simulink model "gm_sampleModel1438_4_sub"  (R2023a)
settings: Solver=VariableStepAuto  StartTime=0.0  StopTime=10.0  RelTol=1e-3
libraries: simulink x1, hdlsllib x1
settings Model: Creator=user1  LastModifiedBy=user1
settings OptimizationCC: BlockReduction=off  ConditionallyExecuteInputs=off
settings DebuggingCC: InheritedTsInSrcMsg=none

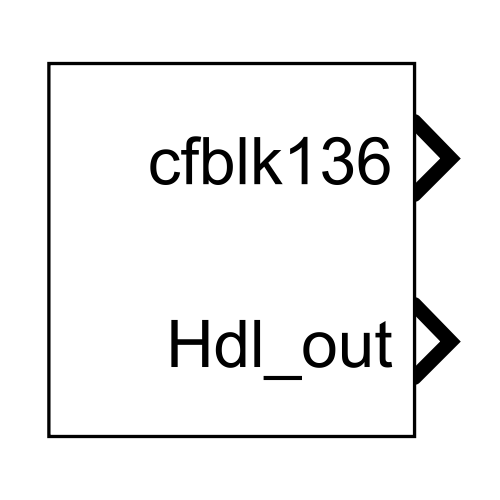
[thumbnail: Simulink's stored preview of the top-level diagram]
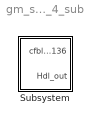
== system gm_sampleModel1438_4_sub ==
  Subsystem : Subsystem

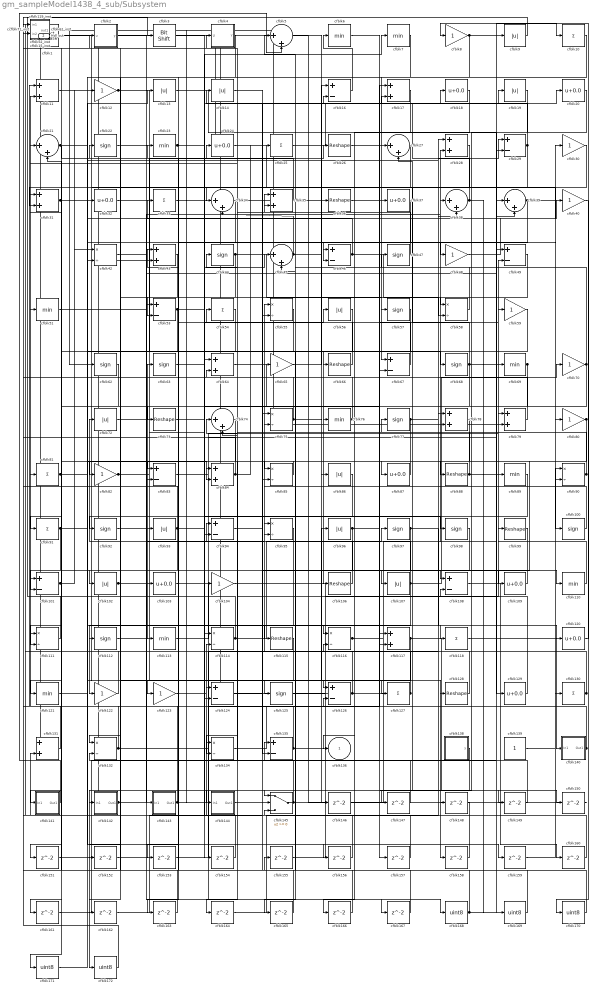
== system gm_sampleModel1438_4_sub/Subsystem ==
  cfblk1 : simulink/Logic and Bit Operations/Detect Decrease  vinit=0.0  OutDataTypeStr=uint8
      settings: LibrarySourceBlock=|
      | hdlsllib/Logic and Bit
      | Operations/Detect
      | Decrease
  cfblk{10,25,33,54,81,91,118,127,130} (9 alike) : Sum  Inputs=+  OutDataTypeStr=uint8
  cfblk{22,44,47,57,62..63,68,77,92,97..98,100,112,125} (14 alike) : Signum
  cfblk{16,29,46,49,53,67,83,94,101,108,124,126,135} (13 alike) : Sum  Inputs=+-  OutDataTypeStr=uint8
  cfblk{9,13..14,19,56,72,86,93,96,102,107} (11 alike) : Abs  OutDataTypeStr=uint8  SaturateOnIntegerOverflow=off
  cfblk{18,20,24,32,37,87,103,109,120,129} (10 alike) : Bias  Bias=0.0  SaturateOnIntegerOverflow=off
  cfblk{8,12,30,40,48,59,65,70,80,82,104,122..123} (13 alike) : Gain  OutDataTypeStr=uint8
  cfblk105_inst : Subsystem
  cfblk{26,36,66,73,88,99,106,115,128} (9 alike) : Reshape
  cfblk{11,17,28,31,35,43,64,78..79,84,117,131} (12 alike) : Sum  OutDataTypeStr=uint8
  cfblk{6..7,23,51,69,76,89,110,113,121} (10 alike) : MinMax  OutDataTypeStr=uint8
  cfblk{42,55,58,75,85,90,95,111,114,116,132,134} (12 alike) : Product  Inputs=*/  OutDataTypeStr=uint8  RndMeth=Zero  SaturateOnIntegerOverflow=on
  cfblk119_inst : Subsystem
  cfblk138 : Subsystem  mask(Counter Free-Running){NumBits=double(16), tsamp=double(-1)}
      mask prompts: NumBits "Simulink:masks:NumberOfBits_MP"; tsamp "Simulink:masks:SampleTime_MP"
      mask help: Simulink:masks:CounterFreeRunning_MD
  cfblk139 : Constant  OutDataTypeStr=uint8  SampleTime=-1
  cfblk140 : Subsystem
  cfblk141 : Subsystem
  cfblk142 : Subsystem
  cfblk143 : Subsystem
  cfblk144 : Subsystem
  cfblk145 : Switch  OutDataTypeStr=uint8  SaturateOnIntegerOverflow=off  InputSameDT=off
  cfblk{146..167} (22 alike) : Delay  SampleTime=1
  cfblk15_inst : Subsystem
  cfblk{168..172} (5 alike) : DataTypeConversion  OutDataTypeStr=uint8  SaturateOnIntegerOverflow=off  RndMeth=Floor
  cfblk2 : Subsystem  mask(Compare To Zero){relop=<=, OutDataTypeStr=uint8, ZeroCross=on}
      mask prompts: relop "Simulink:masks:Operator_MP"; OutDataTypeStr "Simulink:masks:OutputDataType_MP"; ZeroCross "Simulink:masks:EnableZerocrossingDetection_MP"
      mask help: Simulink:masks:CompareToZero_MD
      mask init:
      | OutDataTypeStr = 'uint8';
      | ZeroCross = 'on';
      | blkName = 'sampleModel1438_4_sub/Subsystem/cfblk2';
      | relop = '<=';
      | setValue = 'fixdt(0, 8)';
      mask TypeOptions relop: == | ~= | < | <= | >= | >
      mask TypeOptions OutDataTypeStr: Simulink:masks:uint8 | Simulink:masks:boolean
      mask Callback ZeroCross: sl('zeroCrossEnable', gcbh);
      mask Display: disp([relop,' 0'])
  cfblk{5,21,27,34,38..39,45,74} (8 alike) : Sum  Inputs=|++  OutDataTypeStr=uint8
  cfblk3 : hdlsllib/Logic and Bit Operations/Bit Shift  mode=Shift Left Logical  N=0
  cfblk4 : Subsystem  mask(Detect Fall Nonpositive){vinit=double(0), InputProcessing=Elements as channels (sample based), OutDataTypeStr=uint8}
      mask prompts: vinit "Simulink:masks:InitialCondition_MP"; InputProcessing "Simulink:masks:InputProcessing_MP"; OutDataTypeStr "Simulink:masks:OutputDataType_MP"
      mask help: Simulink:masks:DetectFallNonpositive_MD
      mask init:
      | InputProcessing = 'Elements as channels (sample based)';
      | OutDataTypeStr = 'uint8';
      | vinit = double(0);
      mask TypeOptions InputProcessing: Simulink:masks:ColumnsAsChannelsFrameBased | Simulink:masks:ElementsAsChannelsSampleBased
      mask TypeOptions OutDataTypeStr: Simulink:masks:uint8 | Simulink:masks:boolean
      mask Display: fprintf('U <= 0\n&  NOT\nU/z <= 0')
  cfblk52_inst : Subsystem
  cfblk61_inst : Subsystem
  cfblk71_inst : Subsystem
  cfblk136 : Outport  OutDataTypeStr=uint8  SampleTime=1  VectorParamsAs1DForOutWhenUnconnected=off
  Hdl_out : Outport  Port=2  OutDataTypeStr=uint8  SampleTime=1
  wires:
  cfblk1/1 -> cfblk123/1
  cfblk10/1 -> cfblk67/1
  cfblk100/1 -> cfblk55/1
  cfblk101/1 -> cfblk32/1, cfblk42/1
  cfblk102/1 -> cfblk24/1, cfblk158/1
  cfblk103/1 -> cfblk167/1
  cfblk104/1 -> cfblk108/2
  cfblk105_inst/1(out1) -> cfblk143/1(In1)
  cfblk106/1 -> cfblk72/1
  cfblk107/1 -> cfblk75/2, cfblk70/1, cfblk122/1
  cfblk108/1 -> cfblk160/1
  cfblk109/1 -> cfblk108/1
  cfblk11/1 -> cfblk90/2
  cfblk110/1 -> cfblk49/2
  cfblk111/1 -> cfblk3/1
  cfblk112/1 -> cfblk63/1
  cfblk113/1 -> cfblk79/1
  cfblk114/1 -> cfblk97/1, cfblk11/2
  cfblk115/1 -> cfblk125/1
  cfblk116/1 -> cfblk39/1, cfblk28/2
  cfblk117/1 -> cfblk150/1, cfblk132/1
  cfblk118/1 -> cfblk140/1(In1)
  cfblk119_inst/1(out1) -> cfblk36/1
  cfblk12/1 -> cfblk93/1, cfblk106/1
  cfblk120/1 -> cfblk8/1
  cfblk121/1 -> cfblk28/1
  cfblk122/1 -> cfblk51/1
  cfblk123/1 -> cfblk114/2
  cfblk124/1 -> cfblk18/1
  cfblk125/1 -> cfblk99/1
  cfblk126/1 -> cfblk74/1, cfblk54/1
  cfblk127/1 -> cfblk95/1, Hdl_out/1
  cfblk128/1 -> cfblk61_inst/1(in1)
  cfblk129/1 -> cfblk64/2
  cfblk13/1 -> cfblk129/1
  cfblk130/1 -> cfblk74/2, cfblk45/2
  cfblk131/1 -> cfblk11/1
  cfblk132/1 -> cfblk78/1, cfblk119_inst/1(in1)
  cfblk134/1 -> cfblk37/1
  cfblk135/1 -> cfblk22/1, cfblk17/1
  cfblk138/1(y) -> cfblk172/1
  cfblk139/1 -> cfblk130/1
  cfblk14/1 -> cfblk75/1
  cfblk140/1(Out1) -> cfblk94/1, cfblk64/1
  cfblk141/1(Out1) -> cfblk5/2
  cfblk142/1(Out1) -> cfblk38/1, cfblk95/2
  cfblk143/1(Out1) -> cfblk126/2, cfblk81/1
  cfblk144/1(Out1) -> cfblk55/2
  cfblk145/1 -> cfblk96/1, cfblk14/1
  cfblk146/1 -> cfblk78/2
  cfblk147/1 -> cfblk132/2
  cfblk148/1 -> cfblk145/3
  cfblk149/1 -> cfblk35/1
  cfblk15_inst/1(out1) -> cfblk27/1
  cfblk150/1 -> cfblk1/1
  cfblk151/1 -> cfblk94/2
  cfblk152/1 -> cfblk85/2
  cfblk153/1 -> cfblk116/2
  cfblk154/1 -> cfblk131/2
  cfblk155/1 -> cfblk67/2
  cfblk156/1 -> cfblk105_inst/2(in2)
  cfblk157/1 -> cfblk124/1
  cfblk158/1 -> cfblk83/2
  cfblk159/1 -> cfblk90/1
  cfblk16/1 -> cfblk6/1
  cfblk160/1 -> cfblk52_inst/2(in2)
  cfblk161/1 -> cfblk39/2
  cfblk162/1 -> cfblk114/1
  cfblk163/1 -> cfblk31/1
  cfblk164/1 -> cfblk38/2
  cfblk165/1 -> cfblk43/1
  cfblk166/1 -> cfblk135/1
  cfblk167/1 -> cfblk145/2
  cfblk168/1 -> cfblk9/1, cfblk155/1
  cfblk169/1 -> cfblk2/1(u)
  cfblk17/1 -> cfblk166/1
  cfblk170/1 -> cfblk71_inst/1(in1)
  cfblk171/1 -> cfblk40/1
  cfblk172/1 -> cfblk71_inst/2(in2)
  cfblk18/1 -> cfblk66/1
  cfblk19/1 -> cfblk148/1
  cfblk2/1(y) -> cfblk168/1
  cfblk20/1 -> cfblk58/1
  cfblk21/1 -> cfblk46/2, cfblk126/1, cfblk161/1
  cfblk22/1 -> cfblk103/1
  cfblk23/1 -> cfblk98/1, cfblk7/1
  cfblk24/1 -> cfblk157/1
  cfblk25/1 -> cfblk19/1
  cfblk26/1 -> cfblk128/1
  cfblk27/1 -> cfblk46/1
  cfblk28/1 -> cfblk147/1
  cfblk29/1 -> cfblk31/2, cfblk4/1(U)
  cfblk3/1 -> cfblk76/1
  cfblk30/1 -> cfblk34/1
  cfblk31/1 -> cfblk84/2, cfblk68/1, cfblk13/1
  cfblk32/1 -> cfblk100/1
  cfblk33/1 -> cfblk154/1
  cfblk34/1 -> cfblk153/1
  cfblk35/1 -> cfblk52_inst/1(in1)
  cfblk36/1 -> cfblk149/1
  cfblk37/1 -> cfblk73/1
  cfblk38/1 -> cfblk17/2, cfblk69/1
  cfblk39/1 -> cfblk80/1, cfblk136/1
  cfblk4/1(Y) -> cfblk82/1
  cfblk40/1 -> cfblk170/1
  cfblk42/1 -> cfblk113/1
  cfblk43/1 -> cfblk142/1(In1)
  cfblk44/1 -> cfblk57/1, cfblk124/2
  cfblk45/1 -> cfblk86/1, cfblk34/2
  cfblk46/1 -> cfblk58/2, cfblk33/1
  cfblk47/1 -> cfblk15_inst/1(in1)
  cfblk48/1 -> cfblk30/1
  cfblk49/1 -> cfblk53/2
  cfblk5/1 -> cfblk127/1
  cfblk51/1 -> cfblk115/1
  cfblk52_inst/1(out1) -> cfblk43/2
  cfblk53/1 -> cfblk26/1, cfblk151/1
  cfblk54/1 -> cfblk92/1
  cfblk55/1 -> cfblk141/1(In1)
  cfblk56/1 -> cfblk91/1
  cfblk57/1 -> cfblk165/1
  cfblk58/1 -> cfblk5/1
  cfblk59/1 -> cfblk135/2
  cfblk6/1 -> cfblk48/1
  cfblk61_inst/1(out1) -> cfblk62/1, cfblk146/1
  cfblk62/1 -> cfblk121/1
  cfblk63/1 -> cfblk104/1
  cfblk64/1 -> cfblk117/1
  cfblk65/1 -> cfblk16/1
  cfblk66/1 -> cfblk23/1
  cfblk67/1 -> cfblk35/2
  cfblk68/1 -> cfblk27/2, cfblk107/1, cfblk163/1, cfblk89/1
  cfblk69/1 -> cfblk145/1, cfblk111/2
  cfblk7/1 -> cfblk53/1
  cfblk70/1 -> cfblk88/1, cfblk47/1
  cfblk71_inst/1(out1) -> cfblk79/2, cfblk131/1
  cfblk72/1 -> cfblk49/1
  cfblk73/1 -> cfblk56/1
  cfblk74/1 -> cfblk112/1
  cfblk75/1 -> cfblk119_inst/2(in2), cfblk118/1
  cfblk76/1 -> cfblk44/1, cfblk21/2
  cfblk77/1 -> cfblk29/1, cfblk164/1
  cfblk78/1 -> cfblk87/1
  cfblk79/1 -> cfblk65/1
  cfblk8/1 -> cfblk42/2, cfblk10/1
  cfblk80/1 -> cfblk171/1, cfblk109/1
  cfblk81/1 -> cfblk156/1, cfblk12/1
  cfblk82/1 -> cfblk20/1, cfblk16/2
  cfblk83/1 -> cfblk29/2
  cfblk84/1 -> cfblk61_inst/2(in2), cfblk25/1
  cfblk85/1 -> cfblk83/1
  cfblk86/1 -> cfblk102/1
  cfblk87/1 -> cfblk84/1
  cfblk88/1 -> cfblk21/1, cfblk169/1
  cfblk89/1 -> cfblk144/1(In1)
  cfblk9/1 -> cfblk105_inst/1(in1)
  cfblk90/1 -> cfblk77/1, cfblk85/1
  cfblk91/1 -> cfblk101/2, cfblk116/1
  cfblk92/1 -> cfblk159/1
  cfblk93/1 -> cfblk45/1, cfblk15_inst/2(in2), cfblk101/1
  cfblk94/1 -> cfblk110/1
  cfblk95/1 -> cfblk152/1
  cfblk96/1 -> cfblk117/2, cfblk59/1, cfblk111/1
  cfblk97/1 -> cfblk120/1, cfblk134/2
  cfblk98/1 -> cfblk134/1
  cfblk99/1 -> cfblk162/1

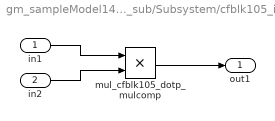
== system gm_sampleModel1438_4_sub/Subsystem/cfblk105_inst ==
  in1 : Inport  OutDataTypeStr=uint8  SampleTime=1
  in2 : Inport  Port=2  OutDataTypeStr=uint8  SampleTime=1
  mul_cfblk105_dotp_mulcomp : Product  Inputs=**  OutDataTypeStr=uint8  SampleTime=1
  out1 : Outport  OutDataTypeStr=uint8  SampleTime=1
  wires:
  in1/1 -> mul_cfblk105_dotp_mulcomp/1
  in2/1 -> mul_cfblk105_dotp_mulcomp/2
  mul_cfblk105_dotp_mulcomp/1 -> out1/1

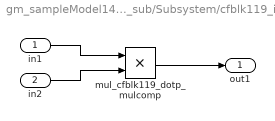
== system gm_sampleModel1438_4_sub/Subsystem/cfblk119_inst ==
  in1 : Inport  OutDataTypeStr=uint8  SampleTime=1
  in2 : Inport  Port=2  OutDataTypeStr=uint8  SampleTime=1
  mul_cfblk119_dotp_mulcomp : Product  Inputs=**  OutDataTypeStr=uint8  SampleTime=1
  out1 : Outport  OutDataTypeStr=uint8  SampleTime=1
  wires:
  in1/1 -> mul_cfblk119_dotp_mulcomp/1
  in2/1 -> mul_cfblk119_dotp_mulcomp/2
  mul_cfblk119_dotp_mulcomp/1 -> out1/1

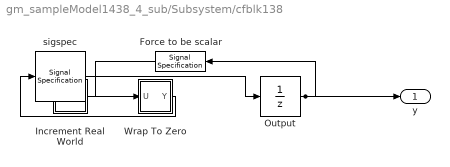
== system gm_sampleModel1438_4_sub/Subsystem/cfblk138 ==
  Force to be scalar : SignalSpecification  DisableCoverage=on  Dimensions=1
  Increment Real World : Subsystem  mask(Real World Value Increment){}
      mask help: Simulink:masks:RealWorldValueIncrement_MD
      mask Display: disp('V++')
  Output : UnitDelay  InitialCondition=0.0  SampleTime=tsamp  HasFrameUpgradeWarning=on
  Wrap To Zero : Subsystem  mask(Wrap To Zero){Threshold=double(65535)}
      mask prompts: Threshold "Simulink:masks:Threshold_MP"
      mask help: Simulink:masks:WrapToZero_MD
  sigspec : SignalSpecification  OutDataTypeStr=uint16  Dimensions=1
  y : Outport  SampleTime=1
  wires:
  Force to be scalar/1 -> Increment Real World/1(u)
  Increment Real World/1(y) -> Wrap To Zero/1(U)
  Output/1 -> Force to be scalar/1, y/1
  Wrap To Zero/1(Y) -> sigspec/1
  sigspec/1 -> Output/1

== system gm_sampleModel1438_4_sub/Subsystem/cfblk140 ==
  In1 : Inport  OutDataTypeStr=uint8  PortDimensions=1  SampleTime=1
  Out1 : Outport  SampleTime=1
  wires:
  In1/1 -> Out1/1

== system gm_sampleModel1438_4_sub/Subsystem/cfblk141 ==
  In1 : Inport  OutDataTypeStr=uint8  PortDimensions=1  SampleTime=1
  Out1 : Outport  SampleTime=1
  wires:
  In1/1 -> Out1/1

== system gm_sampleModel1438_4_sub/Subsystem/cfblk142 ==
  In1 : Inport  OutDataTypeStr=uint8  PortDimensions=1  SampleTime=1
  Out1 : Outport  SampleTime=1
  wires:
  In1/1 -> Out1/1

== system gm_sampleModel1438_4_sub/Subsystem/cfblk143 ==
  In1 : Inport  OutDataTypeStr=uint8  PortDimensions=1  SampleTime=1
  Out1 : Outport  SampleTime=1
  wires:
  In1/1 -> Out1/1

== system gm_sampleModel1438_4_sub/Subsystem/cfblk144 ==
  In1 : Inport  OutDataTypeStr=uint8  PortDimensions=1  SampleTime=1
  Out1 : Outport  SampleTime=1
  wires:
  In1/1 -> Out1/1

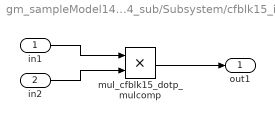
== system gm_sampleModel1438_4_sub/Subsystem/cfblk15_inst ==
  in1 : Inport  OutDataTypeStr=uint8  SampleTime=1
  in2 : Inport  Port=2  OutDataTypeStr=uint8  SampleTime=1
  mul_cfblk15_dotp_mulcomp : Product  Inputs=**  OutDataTypeStr=uint8  SampleTime=1
  out1 : Outport  OutDataTypeStr=uint8  SampleTime=1
  wires:
  in1/1 -> mul_cfblk15_dotp_mulcomp/1
  in2/1 -> mul_cfblk15_dotp_mulcomp/2
  mul_cfblk15_dotp_mulcomp/1 -> out1/1

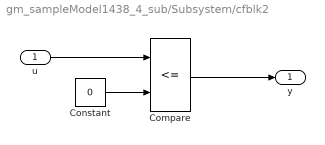
== system gm_sampleModel1438_4_sub/Subsystem/cfblk2 ==
  u : Inport  OutDataTypeStr=uint8  SampleTime=1
  Compare : RelationalOperator  Operator=<=  OutDataTypeStr=fixdt(0, 8)
  Constant : Constant  DisableCoverage=on  Value=0  OutDataTypeStr=Inherit: Inherit via back propagation  SampleTime=-1  PreserveConstantTs=on
  y : Outport  SampleTime=1
  wires:
  u/1 -> Compare/1
  Compare/1 -> y/1
  Constant/1 -> Compare/2

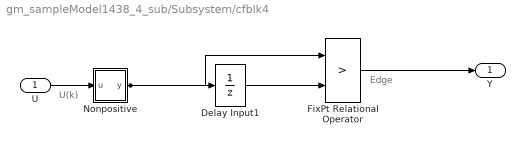
== system gm_sampleModel1438_4_sub/Subsystem/cfblk4 ==
  note: U(k)
  note: Edge
  U : Inport  OutDataTypeStr=uint8  SampleTime=1
  Delay Input1 : UnitDelay  Description=Store in Global RAM  DisableCoverage=on  InitialCondition=vinit  SampleTime=-1  HasFrameUpgradeWarning=on
  FixPt Relational Operator : RelationalOperator  Operator=>  OutDataTypeStr=fixdt(0, 8)  ZeroCross=off  InputSameDT=off
  Nonpositive : Subsystem  mask(Compare To Zero){relop=<=, OutDataTypeStr=boolean, ZeroCross=off}
      mask prompts: relop "Simulink:masks:Operator_MP"; OutDataTypeStr "Simulink:masks:OutputDataType_MP"; ZeroCross "Simulink:masks:EnableZerocrossingDetection_MP"
      mask help: Simulink:masks:CompareToZero_MD
      mask init:
      | OutDataTypeStr = 'boolean';
      | ZeroCross = 'off';
      | blkName = 'sampleModel1438_4_sub/Subsystem/cfblk4/Nonpositive';
      | relop = '<=';
      | setValue = 'boolean';
      mask TypeOptions relop: == | ~= | < | <= | >= | >
      mask TypeOptions OutDataTypeStr: Simulink:masks:uint8 | Simulink:masks:boolean
      mask Callback ZeroCross: sl('zeroCrossEnable', gcbh);
      mask Display: disp([relop,' 0'])
  Y : Outport  SampleTime=1
  wires:
  U/1 -> Nonpositive/1(u)
  Delay Input1/1 -> FixPt Relational Operator/2
  FixPt Relational Operator/1 -> Y/1
  Nonpositive/1(y) -> FixPt Relational Operator/1, Delay Input1/1

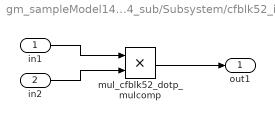
== system gm_sampleModel1438_4_sub/Subsystem/cfblk52_inst ==
  in1 : Inport  OutDataTypeStr=uint8  SampleTime=1
  in2 : Inport  Port=2  OutDataTypeStr=uint8  SampleTime=1
  mul_cfblk52_dotp_mulcomp : Product  Inputs=**  OutDataTypeStr=uint8  SampleTime=1
  out1 : Outport  OutDataTypeStr=uint8  SampleTime=1
  wires:
  in1/1 -> mul_cfblk52_dotp_mulcomp/1
  in2/1 -> mul_cfblk52_dotp_mulcomp/2
  mul_cfblk52_dotp_mulcomp/1 -> out1/1

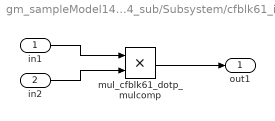
== system gm_sampleModel1438_4_sub/Subsystem/cfblk61_inst ==
  in1 : Inport  OutDataTypeStr=uint8  SampleTime=1
  in2 : Inport  Port=2  OutDataTypeStr=uint8  SampleTime=1
  mul_cfblk61_dotp_mulcomp : Product  Inputs=**  OutDataTypeStr=uint8  SampleTime=1
  out1 : Outport  OutDataTypeStr=uint8  SampleTime=1
  wires:
  in1/1 -> mul_cfblk61_dotp_mulcomp/1
  in2/1 -> mul_cfblk61_dotp_mulcomp/2
  mul_cfblk61_dotp_mulcomp/1 -> out1/1

== system gm_sampleModel1438_4_sub/Subsystem/cfblk71_inst ==
  in1 : Inport  OutDataTypeStr=uint8  SampleTime=1
  in2 : Inport  Port=2  OutDataTypeStr=uint8  SampleTime=1
  mul_cfblk71_dotp_mulcomp : Product  Inputs=**  OutDataTypeStr=uint8  SampleTime=1
  out1 : Outport  OutDataTypeStr=uint8  SampleTime=1
  wires:
  in1/1 -> mul_cfblk71_dotp_mulcomp/1
  in2/1 -> mul_cfblk71_dotp_mulcomp/2
  mul_cfblk71_dotp_mulcomp/1 -> out1/1

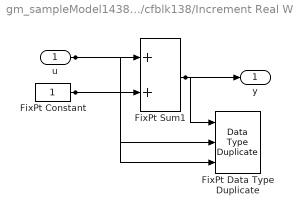
== system gm_sampleModel1438_4_sub/Subsystem/cfblk138/Increment Real World ==
  u : Inport  OutDataTypeStr=uint16  SampleTime=1
  FixPt Constant : Constant  DisableCoverage=on  OutDataTypeStr=Inherit: Inherit via back propagation  SampleTime=-1
  FixPt Data Type Duplicate : DataTypeDuplicate  DisableCoverage=on  NumInputPorts=3
  FixPt Sum1 : Sum  InputSameDT=on  OutDataTypeStr=Inherit: Inherit via back propagation  LockScale=on
  y : Outport  SampleTime=1
  wires:
  u/1 -> FixPt Sum1/1, FixPt Data Type Duplicate/2
  FixPt Constant/1 -> FixPt Sum1/2, FixPt Data Type Duplicate/3
  FixPt Sum1/1 -> FixPt Data Type Duplicate/1, y/1

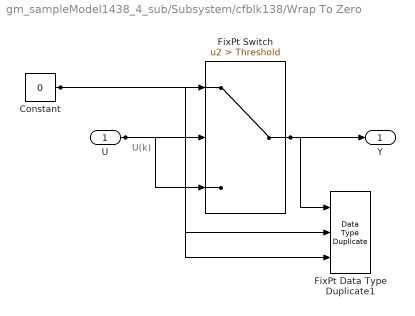
== system gm_sampleModel1438_4_sub/Subsystem/cfblk138/Wrap To Zero ==
  note: U(k)
  U : Inport  OutDataTypeStr=uint16  SampleTime=1
  Constant : Constant  DisableCoverage=on  Value=0  OutDataTypeStr=Inherit: Inherit via back propagation  SampleTime=-1
  FixPt Data Type Duplicate1 : DataTypeDuplicate  DisableCoverage=on  NumInputPorts=3
  FixPt Switch : Switch  Criteria=u2 > Threshold  Threshold=Threshold  OutDataTypeStr=Inherit: Inherit via back propagation  ZeroCross=off  SaturateOnIntegerOverflow=off  InputSameDT=off
  Y : Outport  SampleTime=1
  wires:
  U/1 -> FixPt Switch/3, FixPt Switch/2, FixPt Data Type Duplicate1/2
  Constant/1 -> FixPt Switch/1, FixPt Data Type Duplicate1/3
  FixPt Switch/1 -> FixPt Data Type Duplicate1/1, Y/1

== system gm_sampleModel1438_4_sub/Subsystem/cfblk4/Nonpositive ==
  u : Inport  OutDataTypeStr=uint8  SampleTime=1
  Compare : RelationalOperator  Operator=<=  OutDataTypeStr=boolean  ZeroCross=off
  Constant : Constant  DisableCoverage=on  Value=0  OutDataTypeStr=Inherit: Inherit via back propagation  SampleTime=-1  PreserveConstantTs=on
  y : Outport  SampleTime=1
  wires:
  u/1 -> Compare/1
  Compare/1 -> y/1
  Constant/1 -> Compare/2
